simulink model "Object"  (R2023a)
settings: Solver=VariableStepAuto  StartTime=0.0  StopTime=10.0  RelTol=1e-3
settings Model: Creator=agalimov  LastModifiedBy=agalimov

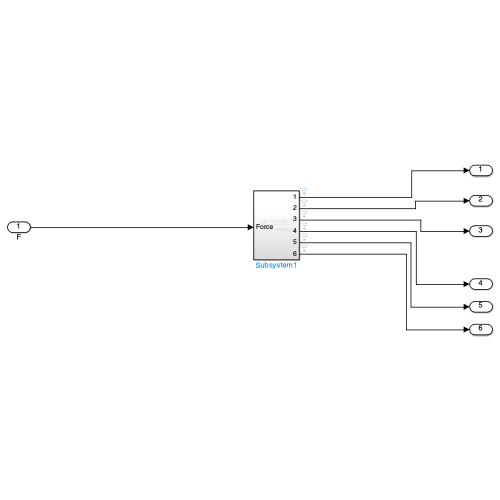
[thumbnail: Simulink's stored preview of the top-level diagram]
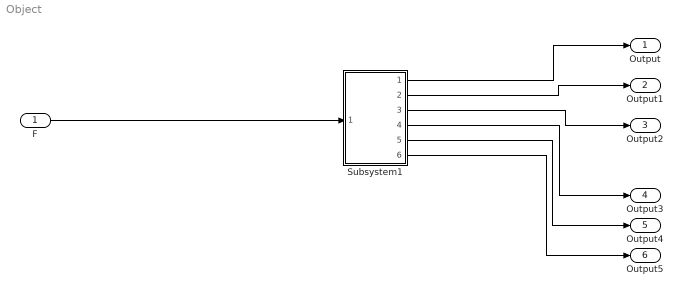
== system Object ==
  F : Inport
  Subsystem1 : Subsystem
  Output : Outport
  Output1 : Outport  Port=2
  Output2 : Outport  Port=3
  Output3 : Outport  Port=4
  Output4 : Outport  Port=5
  Output5 : Outport  Port=6
  wires:
  F/1 -> Subsystem1/1(Force)
  Subsystem1/1(Output) -> Output/1
  Subsystem1/2(Output1) -> Output1/1
  Subsystem1/3(Output2) -> Output2/1
  Subsystem1/4(Output3) -> Output3/1
  Subsystem1/5(Output4) -> Output4/1
  Subsystem1/6(Output5) -> Output5/1

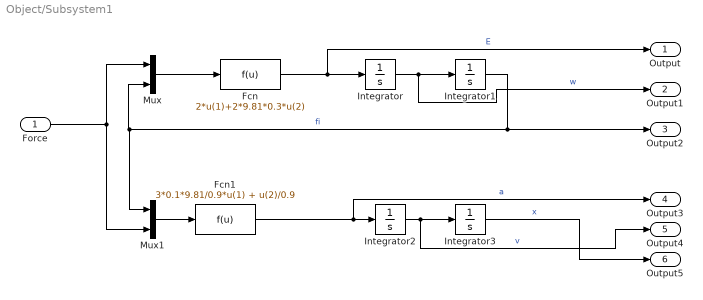
== system Object/Subsystem1 ==
  Force : Inport
  Fcn : Fcn  Expr=2*u(1)+2*9.81*0.3*u(2)
  Fcn1 : Fcn  Expr=3*0.1*9.81/0.9*u(1) + u(2)/0.9
  Integrator : Integrator
  Integrator1 : Integrator  InitialCondition=0.0873
  Integrator2 : Integrator
  Integrator3 : Integrator
  Mux : Mux  Inputs=2
  Mux1 : Mux  Inputs=2
  Output : Outport
  Output1 : Outport  Port=2
  Output2 : Outport  Port=3
  Output3 : Outport  Port=4
  Output4 : Outport  Port=5
  Output5 : Outport  Port=6
  wires:
  Fcn1/1 -> Output3/1, Integrator2/1  "a"
  Integrator3/1 -> Output5/1  "x"
  Integrator2/1 -> Output4/1, Integrator3/1  "v"
  Fcn/1 -> Output/1, Integrator/1  "E"
  Force/1 -> Mux1/2, Mux/1
  Integrator/1 -> Output1/1, Integrator1/1  "w"
  Integrator1/1 -> Mux1/1, Mux/2, Output2/1  "fi"
  Mux1/1 -> Fcn1/1
  Mux/1 -> Fcn/1
